simulink model "control_sys_2"  (R2019b)
settings: Solver=VariableStepAuto  StartTime=0.0  StopTime=10.0  RelTol=1e-3
values from neighbouring files (symbols this model uses):
  A = A*(v_phi(k,i)*s^i)    [Roberts_Q_design.m]    (also in main_fmincon.m = []; rocket_model.m = [0,1,0,0,0,0; ss_model.mat = [0  0; 1  0]; verif.m = [0,1;0,0])
  B = B*(s-alpha(i))    [Roberts_Q_design.m]    (also in controller_design.m = B*C(2); main_yp_fminunc.m = B*C(2); rocket_controllerdesign.m = B*C(2); rocket_controllerdesign_z.m = B*C(2))
  C = [0,1]    [controller_design.m]    (also in main_yp_fminunc.m; rocket_controllerdesign.m; rocket_controllerdesign_z.m; rocket_model.m = eye(6))
  K = minreal(Q/(1+Q*P))    [cost.m]    (also in cost_LQ.m = tf((conv(denQ{1},numK0{1})+conv(numQ{1},den_sys{1})),(conv(d; cost_con.m = tf((conv(denQ{1},numK0{1})+conv(numQ{1},den_sys{1})),(conv(d; cost_disturb.m = tf((conv(denQ{1},numK0{1})+conv(numQ{1},den_sys{1})),(conv(d; fminunc_LQ.m = tf((conv(denQ{1},numK0{1})+conv(numQ{1},den_sys{1})),(conv(d)
  L = lqe(A,G,C,Qe,Re)    [controller_design.m]    (also in main_yp_fminunc.m; rocket_controllerdesign.m; rocket_controllerdesign_z.m; rocket_model.m)
settings Model: Creator=alice  LastModifiedBy=bia
settings SFSimCC: CustomCodeUndefinedFunction=UseInterfaceOnly

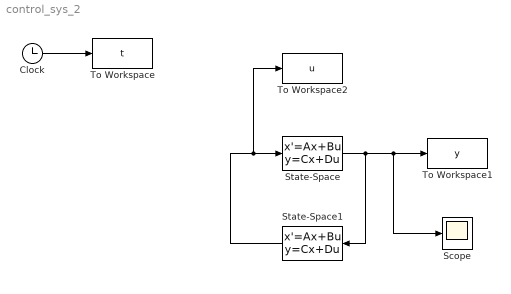
== system control_sys_2 ==
  Clock : Clock
  Scope : Scope
  State-Space : StateSpace  A=A  B=B  C=C  D=0  InitialCondition=0
  State-Space1 : StateSpace  A=A-B*K-L*C  B=L  C=-K  D=0  InitialCondition=0
  To Workspace : ToWorkspace  VariableName=t  SampleTime=-1
  To Workspace1 : ToWorkspace  VariableName=y  SampleTime=-1
  To Workspace2 : ToWorkspace  VariableName=u  SampleTime=-1
  wires:
  Clock/1 -> To Workspace/1
  State-Space/1 -> State-Space1/1, Scope/1, To Workspace1/1
  State-Space1/1 -> To Workspace2/1, State-Space/1
